simulink model "smithpre"  (R2023b)
settings: Solver=VariableStepAuto  StartTime=0.0  StopTime=70  RelTol=1e-3
settings Model: Creator=86189  LastModifiedBy=86189

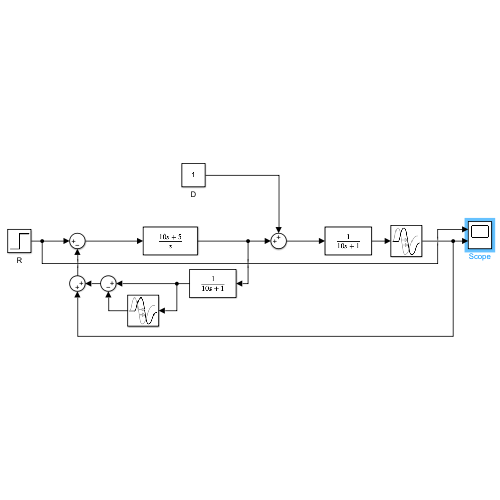
[thumbnail: Simulink's stored preview of the top-level diagram]
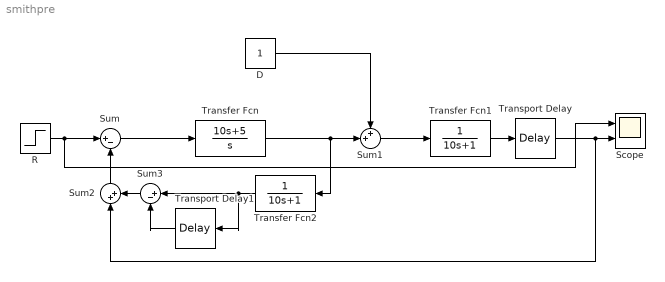
== system smithpre ==
  D : Constant
  R : Step  SampleTime=0
  Scope : Scope  NumInputPorts=2
  Sum : Sum  Inputs=|+-
  Sum1 : Sum  Inputs=++|
  Sum2 : Sum  Inputs=|++
  Sum3 : Sum  Inputs=|+-
  Transfer Fcn : TransferFcn  Numerator=[10 5]  Denominator=[1 0]
  Transfer Fcn1 : TransferFcn  Denominator=[10 1]
  Transfer Fcn2 : TransferFcn  Denominator=[10 1]
  Transport Delay : TransportDelay  DelayTime=10
  Transport Delay1 : TransportDelay  DelayTime=10
  wires:
  Transfer Fcn/1 -> Sum1/2, Transfer Fcn2/1
  Sum1/1 -> Transfer Fcn1/1
  Transfer Fcn1/1 -> Transport Delay/1
  Sum/1 -> Transfer Fcn/1
  Sum2/1 -> Sum/2
  Transport Delay/1 -> Sum2/1, Scope/2
  R/1 -> Scope/1, Sum/1
  D/1 -> Sum1/1
  Sum3/1 -> Sum2/2
  Transfer Fcn2/1 -> Transport Delay1/1, Sum3/1
  Transport Delay1/1 -> Sum3/2
